simulink model "USMcontrolSystem"  (R2017a)
settings: Solver=FixedStepAuto  StartTime=0.0  StopTime=300  FixedStep=0.01666  RelTol=1e-3
values from neighbouring files (symbols this model uses):
  modelParams = load('usm_params.mat')    [vortex_initializeSimulation.m]
  q_IC = zeros(1,8)    [vortexParameters.m]
  T_cm_cb = [rotationX(pi), [0.09 0 0]'; zeros(1,3), 1]    [vortexParameters.m]
  T_head_front = [rotationX(pi), zeros(3,1); zeros(1,3), 1]    [vortexParameters.m]
  T_I_vx = eye(4)    [vortexParameters.m]
  T_tail_back = [rotationZ(pi) * rotationX(pi), [0.105,0,0]'; zeros(1,3), 1]    [vortexParameters.m]
  T_vx_cm_IC = [rotationZ(pi), [0.240, 0, -180]'; zeros(1,3),1]    [vortexParameters.m]
  T_vx_head_IC = [rotationZ(pi), [-1.371,0,-180]'; zeros(1,3), 1]    [vortexParameters.m]
  T_vx_tail_IC = [eye(3), [1.817,0,-180]'; zeros(1,3), 1]    [vortexParameters.m]
undefined symbols (not defined in the file or in its folder): Ke_D, Ke_P, waypoints
undefined symbols (not defined in the file): thrustAlloc
libraries: powerlib_meascontrol x1, Vortex x1
settings Model: Creator=jorgesv  LastModifiedBy=bjorhho

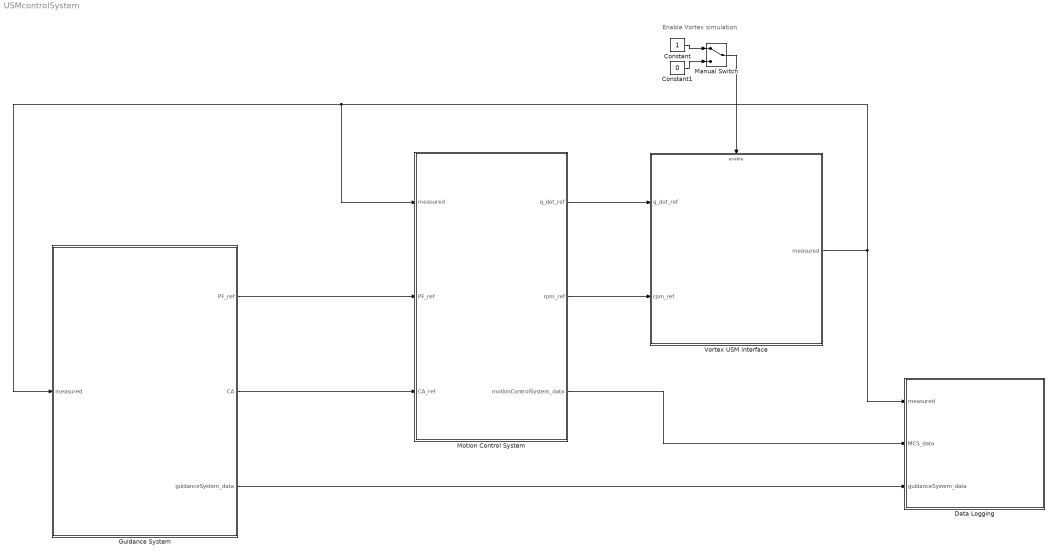
== system USMcontrolSystem ==
  note: Enable Vortex simulation
  Constant : Constant
  Constant1 : Constant  Value=0
  Data Logging : Subsystem
  Guidance System : Subsystem
  Manual Switch : ManualSwitch
  Motion Control System : Subsystem
  Vortex USM interface : Subsystem  TreatAsAtomicUnit=on  mask{T_vx_head_IC=T_vx_head_IC, T_vx_tail_IC=T_vx_tail_IC, q_IC=q_IC, T_0_vx=T_I_vx, T_head_front=T_head_front, T_tail_back=T_tail_back}
      mask prompts: T_vx_head_IC "Transformation from Vortex frame to head module frame"; T_vx_tail_IC "Tronsformation from Vortex frame to tail module frame"; q_IC "Joint positions"; T_0_vx "Transformation from inertial frame to Vortex frame"; T_head_front "Transformation from head module frame to front frame"; T_tail_back "Transformation from tail module frame to back frame"
      settings: MinAlgLoopOccurrences=on
  wires:
  Manual Switch/1 -> Vortex USM interface/Enable
  Constant/1 -> Manual Switch/1
  Constant1/1 -> Manual Switch/2
  Vortex USM interface/1(measured) -> Data Logging/1(measured), Guidance System/1(measured), Motion Control System/1(measured)
  Guidance System/3(guidanceSystem_data) -> Data Logging/3(guidanceSystem_data)
  Guidance System/1(PF_ref) -> Motion Control System/2(PF_ref)
  Motion Control System/2(rpm_ref) -> Vortex USM interface/2(rpm_ref)
  Motion Control System/1(q_dot_ref) -> Vortex USM interface/1(q_dot_ref)
  Motion Control System/3(motionControlSystem_data) -> Data Logging/2(MCS_data)
  Guidance System/2(CA) -> Motion Control System/3(CA_ref)

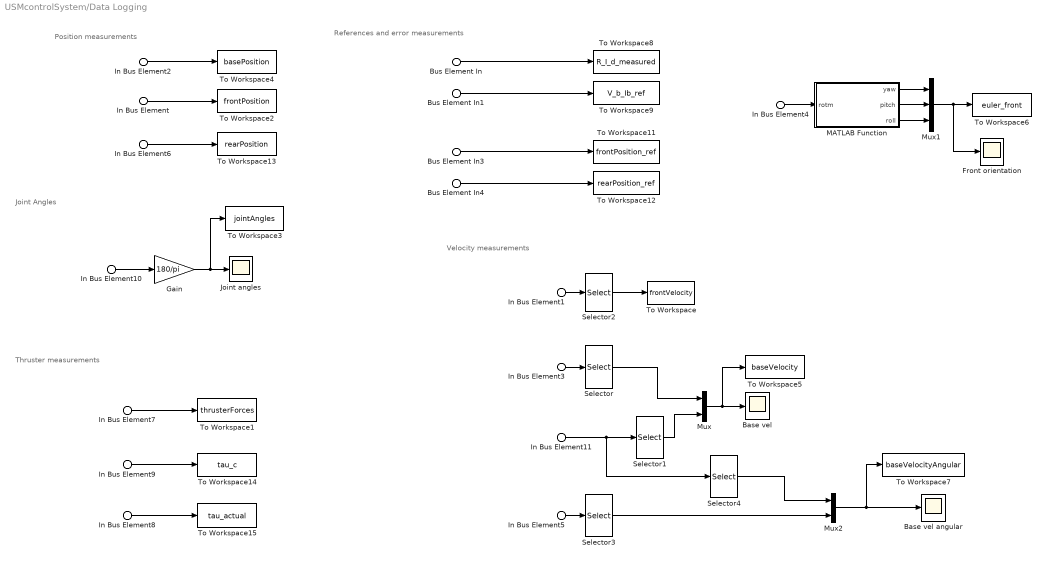
== system USMcontrolSystem/Data Logging ==
  note: References and error measurements
  note: Thruster measurements
  note: Velocity measurements
  note: Position measurements
  note: Joint Angles
  In Bus Element1 : Inport  PortName=measured  Element=V_If_f
  In Bus Element3 : Inport  PortName=measured  Element=V_Ib_b
  In Bus Element5 : Inport  PortName=measured  Element=V_Ib_b
  In Bus Element : Inport  PortName=measured  Element=p_I_f
  In Bus Element2 : Inport  PortName=measured  Element=p_I_b
  In Bus Element4 : Inport  PortName=measured  Element=R_I_f
  In Bus Element6 : Inport  PortName=measured  Element=p_I_r
  In Bus Element10 : Inport  PortName=measured  Element=q_m
  In Bus Element7 : Inport  Port=2  PortName=MCS_data  Element=f_thr
  In Bus Element8 : Inport  Port=2  PortName=MCS_data  Element=actualThrust
  In Bus Element9 : Inport  Port=2  PortName=MCS_data  Element=tau_c
  In Bus Element11 : Inport  Port=2  PortName=MCS_data  Element=V_b_Ib_tilde
  Bus Element In : Inport  Port=3  PortName=guidanceSystem_data  Element=R_I_d
  Bus Element In1 : Inport  Port=3  PortName=guidanceSystem_data  Element=V_b_Ib_tilde
  Bus Element In3 : Inport  Port=3  PortName=guidanceSystem_data  Element=pf_ref
  Bus Element In4 : Inport  Port=3  PortName=guidanceSystem_data  Element=pr_ref
  Base vel : Scope
  Base vel angular : Scope
  Front orientation : Scope
  Gain : Gain  Gain=180/pi
  Joint angles : Scope
  MATLAB Function : MATLAB Function  TreatAsAtomicUnit=on
  Mux : Mux  Inputs=2
  Mux1 : Mux  Inputs=3
  Mux2 : Mux  Inputs=2
  Selector : Selector  InputPortWidth=6  IndexOptions=Index vector (dialog)  Indices=1:3  OutputSizes=1
  Selector1 : Selector  InputPortWidth=6  IndexOptions=Index vector (dialog)  Indices=1:3  OutputSizes=1
  Selector2 : Selector  InputPortWidth=6  IndexOptions=Index vector (dialog)  Indices=1:3  OutputSizes=1
  Selector3 : Selector  InputPortWidth=6  IndexOptions=Index vector (dialog)  Indices=4:6  OutputSizes=1
  Selector4 : Selector  InputPortWidth=6  IndexOptions=Index vector (dialog)  Indices=4:6  OutputSizes=1
  To Workspace : ToWorkspace  VariableName=frontVelocity  SaveFormat=Timeseries  SampleTime=-1
  To Workspace1 : ToWorkspace  VariableName=thrusterForces  SaveFormat=Timeseries  SampleTime=-1
  To Workspace11 : ToWorkspace  VariableName=frontPosition_ref  SaveFormat=Timeseries  SampleTime=-1
  To Workspace12 : ToWorkspace  VariableName=rearPosition_ref  SaveFormat=Timeseries  SampleTime=-1
  To Workspace13 : ToWorkspace  VariableName=rearPosition  SaveFormat=Timeseries  SampleTime=-1
  To Workspace14 : ToWorkspace  VariableName=tau_c  SaveFormat=Timeseries  SampleTime=-1
  To Workspace15 : ToWorkspace  VariableName=tau_actual  SaveFormat=Timeseries  SampleTime=-1
  To Workspace2 : ToWorkspace  VariableName=frontPosition  SaveFormat=Timeseries  SampleTime=-1
  To Workspace3 : ToWorkspace  VariableName=jointAngles  SaveFormat=Timeseries  SampleTime=-1
  To Workspace4 : ToWorkspace  VariableName=basePosition  SaveFormat=Timeseries  SampleTime=-1
  To Workspace5 : ToWorkspace  VariableName=baseVelocity  SaveFormat=Timeseries  SampleTime=-1
  To Workspace6 : ToWorkspace  VariableName=euler_front  SaveFormat=Timeseries  SampleTime=-1
  To Workspace7 : ToWorkspace  VariableName=baseVelocityAngular  SaveFormat=Timeseries  SampleTime=-1
  To Workspace8 : ToWorkspace  VariableName=R_I_d_measured  SaveFormat=Timeseries  SampleTime=-1
  To Workspace9 : ToWorkspace  VariableName=V_b_Ib_ref  SaveFormat=Timeseries  SampleTime=-1
  wires:
  In Bus Element1/1 -> Selector2/1
  In Bus Element3/1 -> Selector/1
  In Bus Element8/1 -> To Workspace15/1
  Selector/1 -> Mux/1
  Selector2/1 -> To Workspace/1
  Gain/1 -> To Workspace3/1, Joint angles/1
  Mux/1 -> To Workspace5/1, Base vel/1
  In Bus Element4/1 -> MATLAB Function/1(rotm)
  MATLAB Function/1(yaw) -> Mux1/1
  MATLAB Function/2(pitch) -> Mux1/2
  MATLAB Function/3(roll) -> Mux1/3
  Mux1/1 -> Front orientation/1, To Workspace6/1
  In Bus Element/1 -> To Workspace2/1
  In Bus Element2/1 -> To Workspace4/1
  Selector1/1 -> Mux/2
  Mux2/1 -> To Workspace7/1, Base vel angular/1
  In Bus Element5/1 -> Selector3/1
  In Bus Element11/1 -> Selector4/1, Selector1/1
  Bus Element In/1 -> To Workspace8/1
  Bus Element In1/1 -> To Workspace9/1
  Bus Element In3/1 -> To Workspace11/1
  Bus Element In4/1 -> To Workspace12/1
  In Bus Element6/1 -> To Workspace13/1
  Selector4/1 -> Mux2/1
  Selector3/1 -> Mux2/2
  In Bus Element7/1 -> To Workspace1/1
  In Bus Element9/1 -> To Workspace14/1
  In Bus Element10/1 -> Gain/1

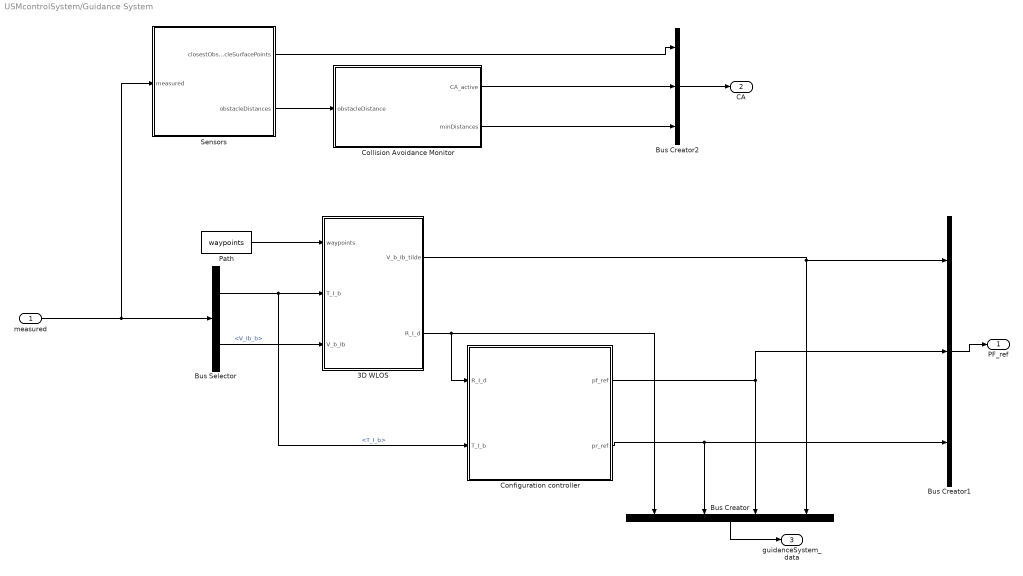
== system USMcontrolSystem/Guidance System ==
  measured : Inport
  3D WLOS : MATLAB Function  TreatAsAtomicUnit=on
  Bus Creator : BusCreator  Inputs=4
  Bus Creator1 : BusCreator  Inputs=3
  Bus Creator2 : BusCreator  Inputs=3
  Bus Selector : BusSelector  OutputSignals=T_I_b,V_Ib_b
  Collision Avoidance Monitor : MATLAB Function  TreatAsAtomicUnit=on
  Configuration controller : MATLAB Function  TreatAsAtomicUnit=on
  Path : Constant  Value=waypoints  VectorParams1D=off
  Sensors : Subsystem
  PF_ref : Outport
  CA : Outport  Port=2
  guidanceSystem_data : Outport  Port=3
  wires:
  Path/1 -> 3D WLOS/1(waypoints)
  3D WLOS/2(R_I_d) -> Configuration controller/1(R_I_d), Bus Creator/1
  Configuration controller/1(pf_ref) -> Bus Creator1/2, Bus Creator/3
  Configuration controller/2(pr_ref) -> Bus Creator/2, Bus Creator1/3
  Bus Creator/1 -> guidanceSystem_data/1
  Bus Creator1/1 -> PF_ref/1
  measured/1 -> Sensors/1(measured), Bus Selector/1
  Bus Selector/1 -> Configuration controller/2(T_I_b), 3D WLOS/2(T_I_b)  "<T_I_b>"
  Bus Selector/2 -> 3D WLOS/3(V_b_Ib)  "<V_Ib_b>"
  Sensors/2(obstacleDistances) -> Collision Avoidance Monitor/1(obstacleDistance)
  Collision Avoidance Monitor/1(CA_active) -> Bus Creator2/2
  Sensors/1(closestObstacleSurfacePoints) -> Bus Creator2/1
  Bus Creator2/1 -> CA/1
  Collision Avoidance Monitor/2(minDistances) -> Bus Creator2/3
  3D WLOS/1(V_b_Ib_tilde) -> Bus Creator/4, Bus Creator1/1

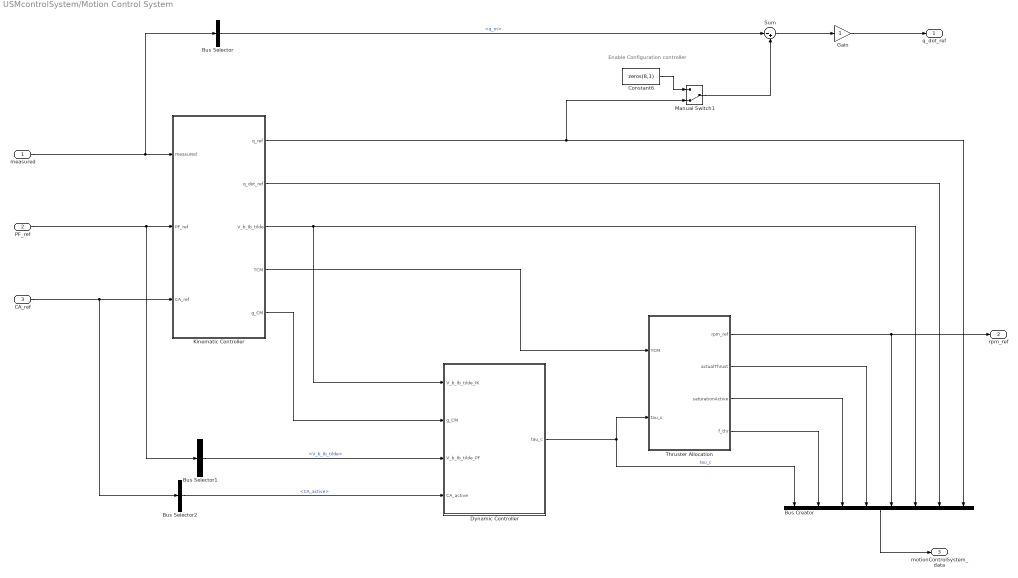
== system USMcontrolSystem/Motion Control System ==
  note: Enable Configuration controller
  measured : Inport
  PF_ref : Inport  Port=2
  CA_ref : Inport  Port=3
  Bus Creator : BusCreator  Inputs=8
  Bus Selector : BusSelector  OutputSignals=q_m
  Bus Selector1 : BusSelector  OutputSignals=V_b_Ib_tilde
  Bus Selector2 : BusSelector  OutputSignals=CA_active
  Constant6 : Constant  Value=zeros(8,1)
  Dynamic Controller : Subsystem
  Gain : Gain
  Kinematic Controller : Subsystem
  Manual Switch1 : ManualSwitch  CurrentSetting=0
  Sum : Sum  Inputs=|-+
  Thruster Allocation : Subsystem  mask{W=thrustAlloc.W_thr, Q_inv=thrustAlloc.Q_thr_inv, mode=thrustAlloc.mode}
      mask prompts: W "Thruster weights"; Q_inv "Pseudoinverse damping matrix (Q_inv)"; mode "Thrust allocation mode"
  q_dot_ref : Outport
  rpm_ref : Outport  Port=2
  motionControlSystem_data : Outport  Port=3
  wires:
  PF_ref/1 -> Bus Selector1/1, Kinematic Controller/2(PF_ref)
  measured/1 -> Bus Selector/1, Kinematic Controller/1(measured)
  Bus Selector/1 -> Sum/1  "<q_m>"
  Dynamic Controller/1(tau_c) -> Thruster Allocation/2(tau_c), Bus Creator/1  "tau_c"
  Thruster Allocation/1(rpm_ref) -> rpm_ref/1, Bus Creator/5
  Bus Creator/1 -> motionControlSystem_data/1
  Thruster Allocation/4(f_thr) -> Bus Creator/2
  Thruster Allocation/3(saturationActive) -> Bus Creator/3
  Thruster Allocation/2(actualThrust) -> Bus Creator/4
  Sum/1 -> Gain/1
  Gain/1 -> q_dot_ref/1
  Manual Switch1/1 -> Sum/2
  Constant6/1 -> Manual Switch1/1
  Kinematic Controller/3(V_b_Ib_tilde) -> Dynamic Controller/1(V_b_Ib_tilde_IK), Bus Creator/6
  CA_ref/1 -> Bus Selector2/1, Kinematic Controller/3(CA_ref)
  Bus Selector2/1 -> Dynamic Controller/4(CA_active)  "<CA_active>"
  Kinematic Controller/2(q_dot_ref) -> Bus Creator/7
  Kinematic Controller/1(q_ref) -> Manual Switch1/2, Bus Creator/8
  Bus Selector1/1 -> Dynamic Controller/3(V_b_Ib_tilde_PF)  "<V_b_Ib_tilde>"
  Kinematic Controller/5(g_CM) -> Dynamic Controller/2(g_CM)
  Kinematic Controller/4(TCM) -> Thruster Allocation/1(TCM)

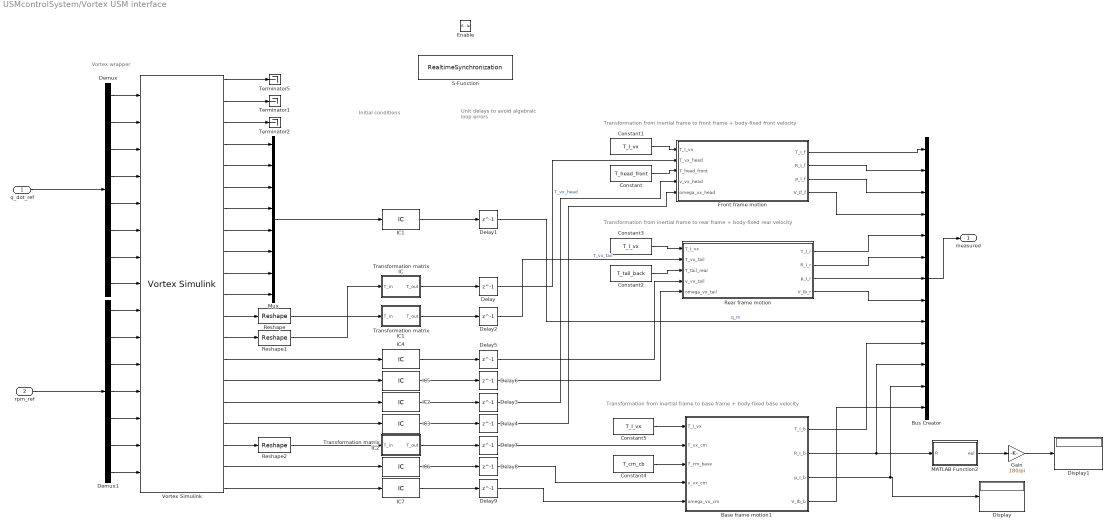
== system USMcontrolSystem/Vortex USM interface ==
  note: Initial conditions
  note: Unit delays to avoid
      | algebraic loop errors
  note: Transformation from inertial frame to front frame + body-fixed front velocity
  note: Vortex wrapper
  note: Transformation from inertial frame to rear frame + body-fixed rear velocity
  note: Transformation from inertial frame to base frame + body-fixed base velocity
  q_dot_ref : Inport  Unit=rad
  rpm_ref : Inport  Port=2  Unit=rpm
  Enable : EnablePort
  Base frame motion1 : MATLAB Function  TreatAsAtomicUnit=on
  Bus Creator : BusCreator  Inputs=13
  Constant : Constant  Value=T_head_front
  Constant1 : Constant  Value=T_I_vx
  Constant2 : Constant  Value=T_tail_back
  Constant3 : Constant  Value=T_I_vx
  Constant4 : Constant  Value=T_cm_cb
  Constant5 : Constant  Value=T_I_vx
  Delay : Delay  DelayLength=1  InitialCondition=T_vx_head_IC
  Delay1 : Delay  DelayLength=1  InitialCondition=q_IC
  Delay2 : Delay  DelayLength=1  InitialCondition=T_vx_tail_IC
  Delay{3..6,8..9} (6 alike) : Delay  DelayLength=1  InitialCondition=[0,0,0]'
  Delay7 : Delay  DelayLength=1  InitialCondition=T_vx_cm_IC
  Demux : Demux  Outputs=8
  Demux1 : Demux  Outputs=7
  Display : Display
  Display1 : Display
  Front frame motion : MATLAB Function  TreatAsAtomicUnit=on
  Gain : Gain  Gain=180/pi
  IC1 : InitialCondition  Value=q_IC
  IC{2..7} (6 alike) : InitialCondition  Value=[0,0,0]'
  MATLAB Function2 : MATLAB Function  TreatAsAtomicUnit=on
  Mux : Mux  Inputs=8
  Rear frame motion : MATLAB Function  TreatAsAtomicUnit=on
  Reshape : Reshape  OutputDimensionality=Customize  OutputDimensions=[4,4]
  Reshape1 : Reshape  OutputDimensionality=Customize  OutputDimensions=[4,4]
  Reshape2 : Reshape  OutputDimensionality=Customize  OutputDimensions=[4,4]
  S-Function : S-Function  FunctionName=RealtimeSynchronization  SFunctionDeploymentMode=off  EnableBusSupport=off
  Terminator1 : Terminator
  Terminator2 : Terminator
  Terminator5 : Terminator
  Transformation matrix IC : Subsystem  mask{T_init=T_vx_head_IC}
      mask prompts: T_init "Initial condition"
      mask DialogControl DescTextVar Prompt: Outputs T_init when T_in is an invalid transformation matrix. Outputs T_in when it is valid.
  Transformation matrix IC1 : Subsystem  mask{T_init=T_vx_tail_IC}
      mask prompts: T_init "Initial condition"
      mask DialogControl DescTextVar Prompt: Outputs T_init when T_in is an invalid transformation matrix. Outputs T_in when it is valid.
  Transformation matrix IC2 : Subsystem  mask{T_init=T_vx_cm_IC}
      mask prompts: T_init "Initial condition"
      mask DialogControl DescTextVar Prompt: Outputs T_init when T_in is an invalid transformation matrix. Outputs T_in when it is valid.
  Vortex Simulink : Vortex/Vortex Simulink  ip='127.0.0.1'  port='736'  path='C:\Users\bjorhho\Google Drive\Skole\NTNU\Masteroppgave\Vortex\Source code\Control System\Vortex-Simulink-interface-velocity.json'  display=image(imread('logo.jpg'), [0, 0, 48, 48]);fprintf('\n\n\nMy Model');port_label('input',1,'q1_cmd');port_label('input',2,'q2_cmd');port_label('input',3,'q3_cmd');port_label('input',4,'q4_cmd');port_label('input',5,'q5_cmd');port_label('input',6,'q6_cmd');port_label('input',7,'q7_cmd');port_label('input',8,'q8_cmd');port_label('input',9,'u1_rpm');port_label('input',10,'u2_rpm');port_label('input',11,'u3_rpm');port_label('input',12,'u4_rpm');port_label('input',13,'u5_rpm');port_label('input',14,'u6_rpm');port_label('input',15,'u7_rpm');port_label('output',1,'Status');port_label('output',2,'Time');port_label('output',3,'FrameIndex');port_label('output',4,'q1');port_label('output',5,'q2');port_label('output',6,'q3');port_label('output',7,'q4');port_label('output',8,'q5');port_label('output',9,'q6');port_label('output',10,'q7');port_label('output',11,'q8');port_label('output',12,'T_vx_tail');port_label('output',13,'T_vx_head');port_label('output',14,'v_vx_tail');port_label('output',15,'w_vx_tail');port_label('output',16,'v_vx_head');port_label('output',17,'w_vx_head');port_label('output',18,'T_vx_cm');port_label('output',19,'v_vx_cm');port_label('output',20,'w_vx_cm');  SynchronizationMechanism=None  WaitVortex=off
      settings: SourceProductName=Vortex
  measured : Outport
  wires:
  Vortex Simulink/17 -> IC3/1
  Vortex Simulink/16 -> IC2/1
  Vortex Simulink/15 -> IC5/1
  Vortex Simulink/14 -> IC4/1
  Reshape/1 -> Transformation matrix IC1/1(T_in)
  Reshape1/1 -> Transformation matrix IC/1(T_in)
  Vortex Simulink/13 -> Reshape1/1
  Vortex Simulink/12 -> Reshape/1
  Vortex Simulink/11 -> Mux/8
  Vortex Simulink/10 -> Mux/7
  Vortex Simulink/9 -> Mux/6
  Vortex Simulink/8 -> Mux/5
  Vortex Simulink/7 -> Mux/4
  Vortex Simulink/6 -> Mux/3
  Vortex Simulink/5 -> Mux/2
  Vortex Simulink/4 -> Mux/1
  Mux/1 -> IC1/1
  Demux1/6 -> Vortex Simulink/14
  Demux1/1 -> Vortex Simulink/9
  Demux1/4 -> Vortex Simulink/12
  Demux1/5 -> Vortex Simulink/13
  Demux1/7 -> Vortex Simulink/15
  Demux1/3 -> Vortex Simulink/11
  Demux1/2 -> Vortex Simulink/10
  Vortex Simulink/1 -> Terminator5/1
  Demux/8 -> Vortex Simulink/8
  Demux/7 -> Vortex Simulink/7
  Demux/6 -> Vortex Simulink/6
  Demux/5 -> Vortex Simulink/5
  Demux/4 -> Vortex Simulink/4
  Demux/3 -> Vortex Simulink/3
  Demux/2 -> Vortex Simulink/2
  Demux/1 -> Vortex Simulink/1
  Vortex Simulink/2 -> Terminator1/1
  Vortex Simulink/3 -> Terminator2/1
  IC1/1 -> Delay1/1
  Delay1/1 -> Bus Creator/9  "q_m"
  Bus Creator/1 -> measured/1
  Constant3/1 -> Rear frame motion/1(T_I_vx)
  Constant2/1 -> Rear frame motion/3(T_tail_rear)
  Constant1/1 -> Front frame motion/1(T_I_vx)
  Front frame motion/1(T_I_f) -> Bus Creator/1
  Front frame motion/2(R_I_f) -> Bus Creator/2
  Front frame motion/4(V_If_f) -> Bus Creator/4
  Delay3/1 -> Front frame motion/4(v_vx_head)
  Constant/1 -> Front frame motion/3(T_head_front)
  Delay/1 -> Front frame motion/2(T_vx_head)  "T_vx_head"
  Delay4/1 -> Front frame motion/5(omega_vx_head)
  Front frame motion/3(p_I_f) -> Bus Creator/3
  MATLAB Function2/1(eul) -> Gain/1
  IC3/1 -> Delay4/1
  IC2/1 -> Delay3/1
  IC5/1 -> Delay6/1
  IC4/1 -> Delay5/1
  Transformation matrix IC1/1(T_out) -> Delay2/1
  Transformation matrix IC/1(T_out) -> Delay/1
  Vortex Simulink/18 -> Reshape2/1
  Vortex Simulink/20 -> IC7/1
  Vortex Simulink/19 -> IC6/1
  Reshape2/1 -> Transformation matrix IC2/1(T_in)
  Transformation matrix IC2/1(T_out) -> Delay7/1
  IC6/1 -> Delay8/1
  IC7/1 -> Delay9/1
  Constant4/1 -> Base frame motion1/3(T_cm_base)
  Constant5/1 -> Base frame motion1/1(T_I_vx)
  Delay7/1 -> Base frame motion1/2(T_vx_cm)
  Delay8/1 -> Base frame motion1/4(v_vx_cm)
  Delay9/1 -> Base frame motion1/5(omega_vx_cm)
  Rear frame motion/4(V_Ib_r) -> Bus Creator/8
  Rear frame motion/3(p_I_r) -> Bus Creator/7
  Rear frame motion/2(R_I_r) -> Bus Creator/6
  Rear frame motion/1(T_I_r) -> Bus Creator/5
  Delay2/1 -> Rear frame motion/2(T_vx_tail)  "T_vx_tail"
  Delay5/1 -> Rear frame motion/4(v_vx_tail)
  Delay6/1 -> Rear frame motion/5(omega_vx_tail)
  Base frame motion1/2(R_I_b) -> Bus Creator/11, MATLAB Function2/1(R)
  Base frame motion1/3(p_I_b) -> Bus Creator/12, Display/1
  Gain/1 -> Display1/1
  rpm_ref/1 -> Demux1/1
  Base frame motion1/1(T_I_b) -> Bus Creator/10
  Base frame motion1/4(V_Ib_b) -> Bus Creator/13
  q_dot_ref/1 -> Demux/1

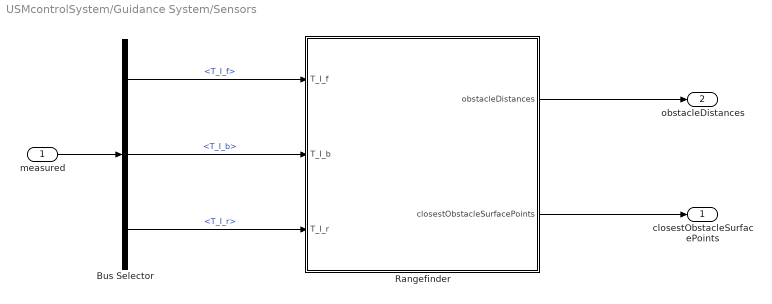
== system USMcontrolSystem/Guidance System/Sensors ==
  measured : Inport
  Bus Selector : BusSelector  OutputSignals=T_I_f,T_I_b,T_I_r
  Rangefinder : MATLAB Function  TreatAsAtomicUnit=on
  closestObstacleSurfacePoints : Outport
  obstacleDistances : Outport  Port=2
  wires:
  measured/1 -> Bus Selector/1
  Bus Selector/1 -> Rangefinder/1(T_I_f)  "<T_I_f>"
  Bus Selector/2 -> Rangefinder/2(T_I_b)  "<T_I_b>"
  Bus Selector/3 -> Rangefinder/3(T_I_r)  "<T_I_r>"
  Rangefinder/1(obstacleDistances) -> obstacleDistances/1
  Rangefinder/2(closestObstacleSurfacePoints) -> closestObstacleSurfacePoints/1

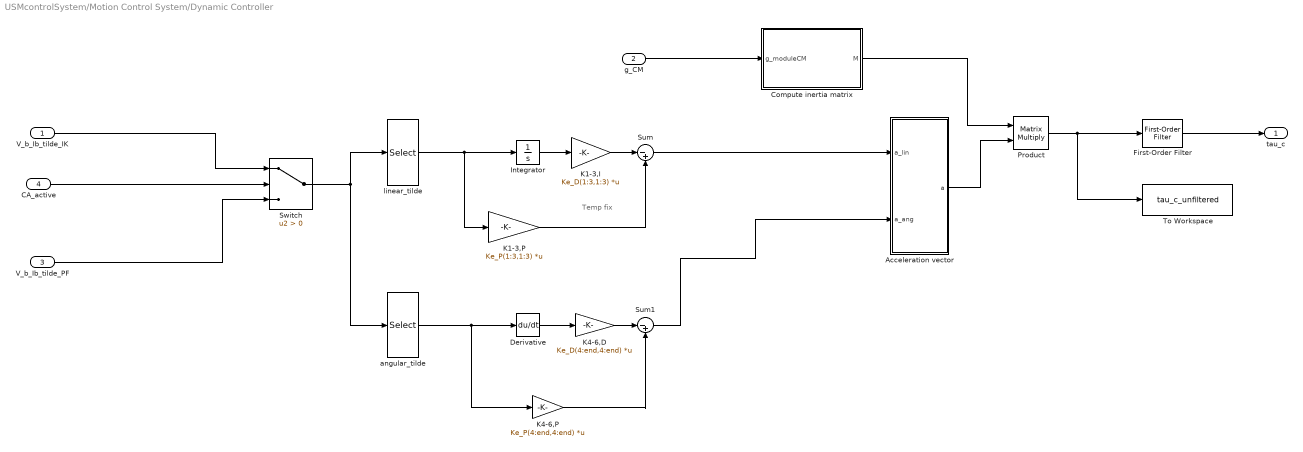
== system USMcontrolSystem/Motion Control System/Dynamic Controller ==
  note: Temp fix
  V_b_Ib_tilde_IK : Inport
  g_CM : Inport  Port=2
  V_b_Ib_tilde_PF : Inport  Port=3
  CA_active : Inport  Port=4
  Acceleration vector : MATLAB Function  TreatAsAtomicUnit=on
  Compute inertia matrix : MATLAB Function  TreatAsAtomicUnit=on
  Derivative : Derivative
  First-Order Filter : powerlib_meascontrol/Filters/First-Order Filter  FilterType=Lowpass  Tc=0.1  Ts=0  Initialize=on  Vac_Init=[0, 0, 60]  Vdc_Init=0  PlotResponse=off  FreqRange="[0,  200,  1]"
      settings: SourceProductName=Simscape Power Systems
  Integrator : Integrator
  K1-3,I : Gain  Gain=Ke_D(1:3,1:3)  Multiplication=Matrix(K*u)
  K1-3,P : Gain  Gain=Ke_P(1:3,1:3)  Multiplication=Matrix(K*u)
  K4-6,D : Gain  Gain=Ke_D(4:end,4:end)  Multiplication=Matrix(K*u)
  K4-6,P : Gain  Gain=Ke_P(4:end,4:end)  Multiplication=Matrix(K*u)
  Product : Product  Multiplication=Matrix(*)
  Sum : Sum  Inputs=|-+
  Sum1 : Sum  Inputs=|-+
  Switch : Switch  Criteria=u2 > Threshold
  To Workspace : ToWorkspace  VariableName=tau_c_unfiltered  SaveFormat=Timeseries  SampleTime=-1
  angular_tilde : Selector  InputPortWidth=6  IndexOptions=Index vector (dialog)  Indices=[4 5 6]  OutputSizes=1
  linear_tilde : Selector  InputPortWidth=6  IndexOptions=Index vector (dialog)  Indices=[1 2 3]  OutputSizes=1
  tau_c : Outport
  wires:
  g_CM/1 -> Compute inertia matrix/1(g_moduleCM)
  Compute inertia matrix/1(M) -> Product/1
  Integrator/1 -> K1-3,I/1
  K1-3,I/1 -> Sum/1
  Derivative/1 -> K4-6,D/1
  K4-6,D/1 -> Sum1/1
  K4-6,P/1 -> Sum1/2
  Sum/1 -> Acceleration vector/1(a_lin)
  Sum1/1 -> Acceleration vector/2(a_ang)
  Acceleration vector/1(a) -> Product/2
  Product/1 -> First-Order Filter/1, To Workspace/1
  First-Order Filter/1 -> tau_c/1
  V_b_Ib_tilde_PF/1 -> Switch/3
  Switch/1 -> angular_tilde/1, linear_tilde/1
  linear_tilde/1 -> K1-3,P/1, Integrator/1
  angular_tilde/1 -> K4-6,P/1, Derivative/1
  K1-3,P/1 -> Sum/2
  CA_active/1 -> Switch/2
  V_b_Ib_tilde_IK/1 -> Switch/1

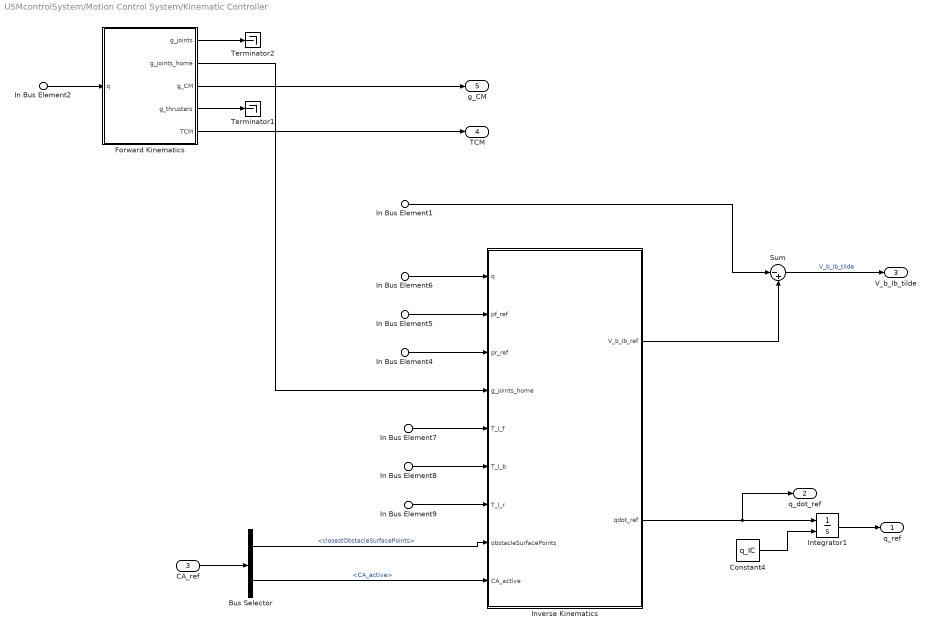
== system USMcontrolSystem/Motion Control System/Kinematic Controller ==
  In Bus Element9 : Inport  PortName=measured  Element=T_I_r
  In Bus Element7 : Inport  PortName=measured  Element=T_I_f
  In Bus Element8 : Inport  PortName=measured  Element=T_I_b
  In Bus Element6 : Inport  PortName=measured  Element=q_m
  In Bus Element2 : Inport  PortName=measured  Element=q_m
  In Bus Element1 : Inport  PortName=measured  Element=V_Ib_b
  In Bus Element4 : Inport  Port=2  PortName=PF_ref  Element=pr_ref
  In Bus Element5 : Inport  Port=2  PortName=PF_ref  Element=pf_ref
  CA_ref : Inport  Port=3
  Bus Selector : BusSelector  OutputSignals=closestObstacleSurfacePoints,CA_active
  Constant4 : Constant  Value=q_IC
  Forward Kinematics : Subsystem
  Integrator1 : Integrator  InitialConditionSource=external  InitialCondition=q_IC
  Inverse Kinematics : MATLAB Function  TreatAsAtomicUnit=on
  Sum : Sum  Inputs=|-+
  Terminator1 : Terminator
  Terminator2 : Terminator
  q_ref : Outport
  q_dot_ref : Outport  Port=2
  V_b_Ib_tilde : Outport  Port=3
  TCM : Outport  Port=4
  g_CM : Outport  Port=5
  wires:
  Forward Kinematics/2(g_joints_home) -> Inverse Kinematics/4(g_joints_home)
  In Bus Element7/1 -> Inverse Kinematics/5(T_I_f)
  In Bus Element8/1 -> Inverse Kinematics/6(T_I_b)
  In Bus Element9/1 -> Inverse Kinematics/7(T_I_r)
  Bus Selector/1 -> Inverse Kinematics/8(obstacleSurfacePoints)  "<closestObstacleSurfacePoints>"
  Constant4/1 -> Integrator1/2
  Inverse Kinematics/2(qdot_ref) -> q_dot_ref/1, Integrator1/1
  Integrator1/1 -> q_ref/1
  CA_ref/1 -> Bus Selector/1
  Bus Selector/2 -> Inverse Kinematics/9(CA_active)  "<CA_active>"
  In Bus Element5/1 -> Inverse Kinematics/2(pf_ref)
  In Bus Element4/1 -> Inverse Kinematics/3(pr_ref)
  In Bus Element6/1 -> Inverse Kinematics/1(q)
  In Bus Element1/1 -> Sum/1
  Inverse Kinematics/1(V_b_Ib_ref) -> Sum/2
  Sum/1 -> V_b_Ib_tilde/1  "V_b_Ib_tilde"
  Forward Kinematics/5(TCM) -> TCM/1
  Forward Kinematics/3(g_CM) -> g_CM/1
  Forward Kinematics/4(g_thrusters) -> Terminator1/1
  Forward Kinematics/1(g_joints) -> Terminator2/1
  In Bus Element2/1 -> Forward Kinematics/1(q)

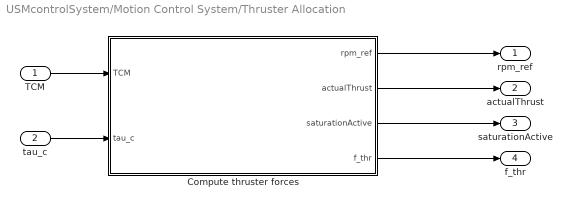
== system USMcontrolSystem/Motion Control System/Thruster Allocation ==
  TCM : Inport
  tau_c : Inport  Port=2
  Compute thruster forces : MATLAB Function  TreatAsAtomicUnit=on
  rpm_ref : Outport
  actualThrust : Outport  Port=2
  saturationActive : Outport  Port=3
  f_thr : Outport  Port=4
  wires:
  Compute thruster forces/1(rpm_ref) -> rpm_ref/1
  TCM/1 -> Compute thruster forces/1(TCM)
  tau_c/1 -> Compute thruster forces/2(tau_c)
  Compute thruster forces/3(saturationActive) -> saturationActive/1
  Compute thruster forces/2(actualThrust) -> actualThrust/1
  Compute thruster forces/4(f_thr) -> f_thr/1

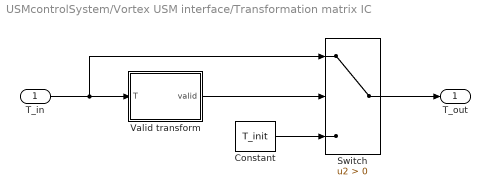
== system USMcontrolSystem/Vortex USM interface/Transformation matrix IC ==
  T_in : Inport
  Constant : Constant  Value=T_init
  Switch : Switch  Criteria=u2 > Threshold
  Valid transform : MATLAB Function  TreatAsAtomicUnit=on
  T_out : Outport
  wires:
  Valid transform/1(valid) -> Switch/2
  T_in/1 -> Switch/1, Valid transform/1(T)
  Constant/1 -> Switch/3
  Switch/1 -> T_out/1

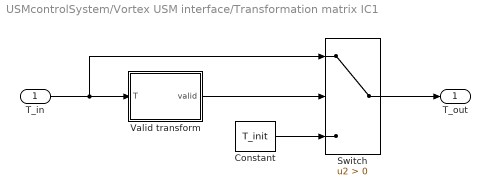
== system USMcontrolSystem/Vortex USM interface/Transformation matrix IC1 ==
  T_in : Inport
  Constant : Constant  Value=T_init
  Switch : Switch  Criteria=u2 > Threshold
  Valid transform : MATLAB Function  TreatAsAtomicUnit=on
  T_out : Outport
  wires:
  Valid transform/1(valid) -> Switch/2
  T_in/1 -> Switch/1, Valid transform/1(T)
  Constant/1 -> Switch/3
  Switch/1 -> T_out/1

== system USMcontrolSystem/Vortex USM interface/Transformation matrix IC2 ==
  T_in : Inport
  Constant : Constant  Value=T_init
  Switch : Switch  Criteria=u2 > Threshold
  Valid transform : MATLAB Function  TreatAsAtomicUnit=on
  T_out : Outport
  wires:
  Switch/1 -> T_out/1
  Constant/1 -> Switch/3
  T_in/1 -> Valid transform/1(T), Switch/1
  Valid transform/1(valid) -> Switch/2

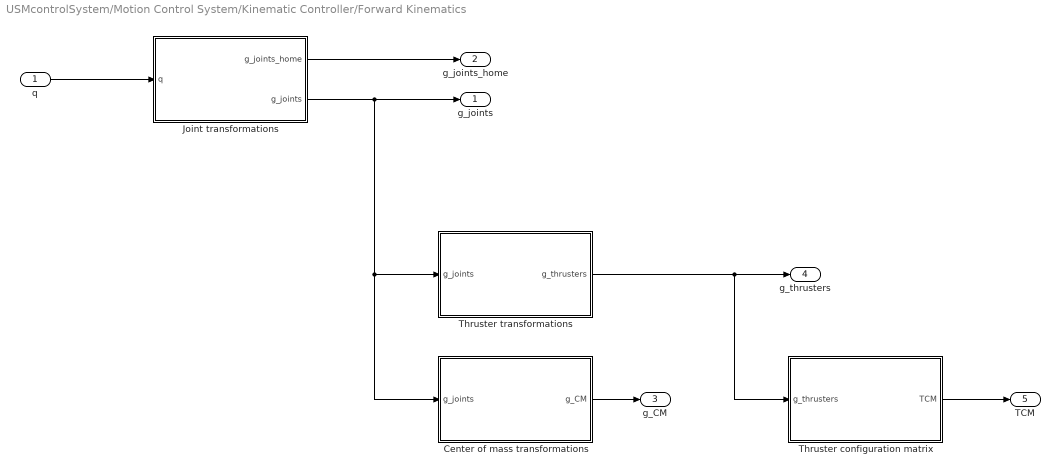
== system USMcontrolSystem/Motion Control System/Kinematic Controller/Forward Kinematics ==
  q : Inport
  Center of mass transformations : MATLAB Function  TreatAsAtomicUnit=on
  Joint transformations : MATLAB Function  TreatAsAtomicUnit=on
  Thruster configuration matrix : MATLAB Function  TreatAsAtomicUnit=on
  Thruster transformations : MATLAB Function  TreatAsAtomicUnit=on
  g_joints : Outport
  g_joints_home : Outport  Port=2
  g_CM : Outport  Port=3
  g_thrusters : Outport  Port=4
  TCM : Outport  Port=5
  wires:
  q/1 -> Joint transformations/1(q)
  Joint transformations/2(g_joints) -> Center of mass transformations/1(g_joints), Thruster transformations/1(g_joints), g_joints/1
  Thruster transformations/1(g_thrusters) -> Thruster configuration matrix/1(g_thrusters), g_thrusters/1
  Center of mass transformations/1(g_CM) -> g_CM/1
  Joint transformations/1(g_joints_home) -> g_joints_home/1
  Thruster configuration matrix/1(TCM) -> TCM/1

== matlab function USMcontrolSystem/Motion Control System/Kinematic Controller/Forward Kinematics/Thruster transformations ==
  data: g_joints input; g_thrusters output; modelParams parameter
function g_thrusters = thrusterTransformations(g_joints, modelParams)
%#codegen

% Compute transformations from the joint frames to the thruster frames

num_thrusters = modelParams.num_thrusters;
thruster_ax = modelParams.thruster_ax;
thruster_pos = modelParams.thruster_pos;
thruster_moduleNumber = modelParams.thruster_moduleNumber;

g_thrusters = calculateThrusterTransformations(g_joints, num_thrusters, thruster_ax, thruster_pos, thruster_moduleNumber);

%NEW
%thruster_rotation = modelParams.thruster_rotation;
%g_thrusters = calculateThrusterTransformations(g_joints, num_thrusters, thruster_rotation, thruster_pos, thruster_moduleNumber);

end

== matlab function USMcontrolSystem/Motion Control System/Kinematic Controller/Forward Kinematics/Joint transformations ==
  data: g_joints_home output; q input; g_joints output; modelParams parameter
function [g_joints_home, g_joints] = jointTransformations(q, modelParams)
%#codegen

% Compute transformations from the back frame to each joint frame and to the front (end-effector) frame

num_joints = modelParams.num_joints;
joint_tr = modelParams.joint_tr;
joint_ax = modelParams.joint_ax;

[g_joints, g_joints_home] = calculateJointTransformations(q, num_joints, joint_tr, joint_ax);

end

== matlab function USMcontrolSystem/Guidance System/Sensors/Rangefinder ==
  data: obstacleDistances output; T_I_f input; closestObstacleSurfacePoints output; T_I_b input; T_I_r input
function [obstacleDistances, closestObstacleSurfacePoints] = distanceToObstacles(T_I_f, T_I_b, T_I_r)
persistent obstacles;
if isempty(obstacles)
    %Obstacle course: (the one used in the thesis)
    %Vertical cyldinders
    R_cyl = 0.5;
    d_circ = sqrt(2);
    c_circ = -7;
    c1 = Cylinder([c_circ + d_circ; -d_circ; -185], [c_circ + d_circ; -d_circ; -175], R_cyl);
    c2 = Cylinder([c_circ + d_circ; d_circ; -185], [c_circ + d_circ; d_circ; -175], R_cyl);

    c3 = Cylinder([c_circ; 0.1; -185], [c_circ; 0.1; -175], R_cyl);

    c4 = Cylinder([c_circ - d_circ; -d_circ; -185], [c_circ - d_circ; -d_circ; -175], R_cyl);
    c5 = Cylinder([c_circ - d_circ; d_circ; -185], [c_circ - d_circ; d_circ; -175], R_cyl);
    %Horizontal cylinders
    c6 = Cylinder([c_circ + d_circ; -d_circ; -180.1], [c_circ + d_circ; d_circ; -180.1], R_cyl);
    c7 = Cylinder([c_circ; 0.1; -179], [c_circ - d_circ; -d_circ + 0.1; -179], R_cyl);
    c8 = Cylinder([c_circ - d_circ; -d_circ; -181], [c_circ - d_circ; d_circ; -181], R_cyl);

    obstacles = {c1, c2, c3, c4, c5, c6, c7, c8};
end

p_I_f = tform2trvec(T_I_f);
p_I_b = tform2trvec(T_I_b);
p_I_r = tform2trvec(T_I_r);

nCAPoints = 3;
%obstacles is a cell array containing obstacles as basic shape objects
nObstacles = numel(obstacles);

obstacleDistances = zeros(nCAPoints, nObstacles);
obstacleSurfacePoints = zeros(3, nCAPoints, nObstacles);
CAPoints = [p_I_f p_I_b p_I_r];

closest = Inf(1, nCAPoints);
closestObstacleSurfacePoints = zeros(3, nCAPoints);
for i = 1:nObstacles
    o = obstacles{i};
    for j = 1:nCAPoints
        obstacleDistances(j, i) = o.distanceTo(CAPoints(:,j));
        obstacleSurfacePoints(:,j,i) = o.closestSurfacePointTo(CAPoints(:,j));
        
        if obstacleDistances(j, i) < closest(j)
            closest(j) = obstacleDistances(j, i);
            closestObstacleSurfacePoints(:,j) = obstacleSurfacePoints(:,j,i);
        end
    end
end

end

== matlab function USMcontrolSystem/Motion Control System/Kinematic Controller/Forward Kinematics/Center of mass transformations ==
  data: g_joints input; g_CM output; modelParams parameter
function g_CM = CMTransformations(g_joints, modelParams)
%#codegen

% Compute transformations from the joint frames to the frames attached to
% center of mass of the modules


num_modules = modelParams.num_modules;
module_cm = modelParams.module_cm;

g_CM = calculateModuleTransformations(g_joints, num_modules, module_cm);

end

== matlab function USMcontrolSystem/Motion Control System/Thruster Allocation/Compute thruster forces ==
  data: TCM input; rpm_ref output; actualThrust output; tau_c input; modelParams parameter; W parameter; saturationActive output; f_thr output; Q_inv parameter; mode parameter
function [rpm_ref, actualThrust, saturationActive, f_thr] = distributeThrusterForces(TCM, tau_c, modelParams, W, Q_inv, mode)
%#codegen

n_thr = modelParams.num_thrusters;
thrusterRPMMapping = modelParams.thrusterRPMMapping;

%W = controlParams.W_thr;
%Q_inv = controlParams.Q_thr_inv;
%mode = controlParams.thrustAllocationMode;




% Calculates the distribution of the thruster forces
W_inv = diag(1./diag(W));

switch mode
    case 0   % Standard damped inverse TCM
        [TCM_inv] = calculateTCMInverse(TCM, Q_inv);
        
        [f_thr] = calculateThrusterForces(TCM_inv, tau_c);
        
    case 1   % Thrust allocation with prioritized linear motion (DOF 1-3)
        [TCM_inv_linear,TCM_inv_angular] = calculateTCMInversePrioritized(TCM, Q_inv);
        
        TCM_inv = [TCM_inv_linear, TCM_inv_angular];
        
        [f_thr] = calculateThrusterForcesPrioritized(TCM(1:3,:),TCM_inv_linear,TCM_inv_angular, tau_c, n_thr);
    
    case 2   % Thrust allocation with inverse TCM using SVD
        TCM_inv = calculateTCMInverseSVD(TCM,0.1);
        [f_thr] = calculateThrusterForces(TCM_inv, tau_c);
        
    otherwise  % Equal to case 0
        [TCM_inv] = calculateTCMInverse(TCM, Q_inv);
        
        [f_thr] = calculateThrusterForces(TCM_inv, tau_c);        
end

actualThrust = TCM * f_thr;

mx = max(thrusterRPMMapping(:,2));
mn = min(thrusterRPMMapping(:,2));


% Min/max force saturation to avoid NaN in the RPM interpolation
saturationActive = ~isempty(find(f_thr > mx,1)) + ~isempty(find(f_thr < mn,1));
f_thr(f_thr > mx) = mx;
f_thr(f_thr < mn) = mn;


% Calculate the required RPM
rpm_ref = interp1(thrusterRPMMapping(:,2), thrusterRPMMapping(:,1), f_thr);

end

== matlab function USMcontrolSystem/Guidance System/Collision Avoidance Monitor ==
  data: obstacleDistance input; CA_active output; minDistances output
function [CA_active, minDistances] = collisionAvoidance(obstacleDistance)

persistent R_active;
if isempty(R_active)
    R_active = 5;
end

n = length(obstacleDistance);
CA_active = 0;
for i = 1:n
    if obstacleDistance <= R_active
        CA_active = 1;
    end
end

minAllowedDistToObstacle = ones(1,n)*0.3;

minDistances = minAllowedDistToObstacle;

%HARD CODED OVERRIDE BECAUSE THIS FUNCTIONALITY IS NOT SUFFICIENTLY
%IMPLEMENTED
%A method for supplying the CA system with a proper desired goal point has
%not been implemeted
CA_active = 0; %PATH FOLLOWING ONLY, i.e IGNORE OBSTACLES
%CA_active = 1; %CA SYSTEM ONLY, i.e IGNORE DESIRED PATH, goal point set in inverse kinematics block
%--------------
end

== matlab function USMcontrolSystem/Motion Control System/Kinematic Controller/Inverse Kinematics ==
  data: q input; pf_ref input; pr_ref input; g_joints_home input; T_I_f input; V_b_Ib_ref output; T_I_b input; T_I_r input; obstacleSurfacePoints input; CA_active input; qdot_ref output; modelParams parameter
function [V_b_Ib_ref, qdot_ref] = simulink_inverseKinematics(q, pf_ref, pr_ref, g_joints_home, T_I_f, T_I_b, T_I_r, obstacleSurfacePoints, CA_active, modelParams)
num_joints = modelParams.num_joints;
bodyTwists = modelParams.bodyTwists;
q_max = modelParams.q_max;
q_min = modelParams.q_min;

% Joint limit avoidance
% Calculating the normalized joint positions
q_normalized = (q - q_min)./(q_max - q_min);
alpha = 0.001;
W_jointLimit = alpha * (2*q_normalized - 1)./((1-q_normalized).^2 .* q_normalized.^2);

%% Calculate geometric Jacobians for the three points on the USM
%Calculate jacobian from base to end-effector
base = 2; %link number
sf = 2*base + 2; %Starting index for joint frames from base module and forward.
g_joints_home_f = g_joints_home(:,:,sf:end);
bodyTwists_f = bodyTwists(:, sf - 1:end);
num_joints_f = num_joints - 2*base;
Jf = calculateGeometricJacobian(g_joints_home_f, num_joints_f, bodyTwists_f);

%Calculate Jacobian from base to rear-end
eb = 2*base + 1; %Ending index for joint frames from base module and backward
num_joints_b = num_joints - num_joints_f;
g_joints_home_b = zeros(4,4,num_joints_b + 1);
for i = 1:eb
    g_joints_home_b(:,:,i) = g_joints_home(:,:, eb + 1 - i);
end
bodyTwists_b = fliplr(bodyTwists(:, 1:eb - 1));
Jr = calculateGeometricJacobian(g_joints_home_b, num_joints_b, bodyTwists_b);

%Calculate jacobian from base to base
Jb = [eye(6), zeros(6,4)];

%% Solve inverse kinematics
if CA_active == 1
    [V_b_Ib_ref, qdot_ref] = CLIK_collisionAvoidance(T_I_f, T_I_b, T_I_r, obstacleSurfacePoints, Jf, Jb, Jr);
else
    [qdot_ref] = CLIK_pathFollowing(Jf, Jr, T_I_f, T_I_r, pf_ref, pr_ref);
    V_b_Ib_ref = zeros(6,1);
end

end

== matlab function USMcontrolSystem/Data Logging/MATLAB Function ==
  data: rotm input; yaw output; pitch output; roll output
function [yaw,pitch,roll] = rotation2Euler(rotm)

eul = rotm2eul(rotm);

yaw = eul(1);
pitch = eul(2);
roll = eul(3);

end

== matlab function USMcontrolSystem/Vortex USM interface/Rear frame motion ==
  data: T_I_r output; R_I_r output; p_I_r output; T_I_vx input; T_vx_tail input; V_Ib_r output; T_tail_rear input; v_vx_tail input; omega_vx_tail input
function [T_I_r, R_I_r, p_I_r, V_Ib_r] = rearFrameMotion(T_I_vx, T_vx_tail, T_tail_rear, v_vx_tail, omega_vx_tail)
% Calculates the linear and angular velocity of the back frame relative to
% the inertial frame I, expressed in the back frame
% Assumption: No relative motion between the Vortex frame, F_vx, and the
% inertial frame, F_I

T_vx_b = T_vx_tail * T_tail_rear;
T_I_r = T_I_vx * T_vx_b;

R_vx_t = tform2rotm(T_vx_tail);
R_vx_b = tform2rotm(T_vx_b);
R_I_r = tform2rotm(T_I_r);
p_I_r = tform2trvec(T_I_r);


p_tb_t = tform2trvec(T_tail_rear);  % Vector from tail (t) to back (b) frame expressed in tail frame

v_Ib_b = R_vx_b' * (v_vx_tail + skew(omega_vx_tail) * R_vx_t * p_tb_t);
    
omega_Ib_b = R_vx_b' * omega_vx_tail;


V_Ib_r = [v_Ib_b; omega_Ib_b];

end

== matlab function USMcontrolSystem/Vortex USM interface/Front frame motion ==
  data: T_I_f output; R_I_f output; p_I_f output; T_I_vx input; T_vx_head input; V_If_f output; T_head_front input; v_vx_head input; omega_vx_head input
function [T_I_f, R_I_f, p_I_f, V_If_f] = frontFrameMotion(T_I_vx, T_vx_head, T_head_front, v_vx_head, omega_vx_head)
% Calculates the linear and angular velocity of the back frame relative to
% the inertial frame I, expressed in the back frame
% Assumption: No relative motion between the Vortex frame, F_vx, and the
% inertial frame, F_I

T_vx_f = T_vx_head * T_head_front;
T_I_f = T_I_vx * T_vx_f;

R_vx_h = tform2rotm(T_vx_head);
R_vx_f = tform2rotm(T_vx_f);
R_I_f = tform2rotm(T_I_f);
p_I_f = tform2trvec(T_I_f);


p_hf_h = tform2trvec(T_head_front);  % Vector from head (h) to front (f) frame expressed in head frame

v_If_f = R_vx_f' * (v_vx_head + skew(omega_vx_head) * R_vx_h * p_hf_h);
    
omega_If_f = R_vx_f' * omega_vx_head;


V_If_f = [v_If_f; omega_If_f];

end

== matlab function USMcontrolSystem/Vortex USM interface/Transformation matrix IC/Valid transform ==
  data: T input; valid output boolean
function valid = fcn(T)

valid = valid_tform(T);

== matlab function USMcontrolSystem/Vortex USM interface/Transformation matrix IC1/Valid transform ==
  data: T input; valid output boolean
function valid = fcn(T)

valid = valid_tform(T);

== matlab function USMcontrolSystem/Vortex USM interface/Base frame motion1 ==
  data: T_I_b output; R_I_b output; p_I_b output; T_I_vx input; T_vx_cm input; V_Ib_b output; T_cm_base input; v_vx_cm input; omega_vx_cm input
function [T_I_b, R_I_b, p_I_b, V_Ib_b] = baseFrameMotion(T_I_vx, T_vx_cm, T_cm_base, v_vx_cm, omega_vx_cm)
% Calculates the linear and angular velocity of the back frame relative to
% the inertial frame I, expressed in the back frame
% Assumption: No relative motion between the Vortex frame, F_vx, and the
% inertial frame, F_I

T_vx_b = T_vx_cm * T_cm_base;
T_I_b = T_I_vx * T_vx_b;

R_vx_c = tform2rotm(T_vx_cm);
R_vx_b = tform2rotm(T_vx_b);
R_I_b = tform2rotm(T_I_b);
p_I_b = tform2trvec(T_I_b);


p_cb_c = tform2trvec(T_cm_base);  % Vector from center module (c) to base (b) frame expressed in center module frame

v_Ib_b = R_vx_b' * (v_vx_cm + skew(omega_vx_cm) * R_vx_c * p_cb_c);
    
omega_Ib_b = R_vx_b' * omega_vx_cm;


V_Ib_b = [v_Ib_b; omega_Ib_b];

end

== matlab function USMcontrolSystem/Guidance System/3D WLOS ==
  data: waypoints input; V_b_Ib_tilde output; R_I_d output; T_I_b input; V_b_Ib input; delta parameter
function [V_b_Ib_tilde, R_I_d]  = simulink_WLOS(waypoints, T_I_b, V_b_Ib, delta)

[V_b_Ib_tilde, R_I_d] = WLOS(waypoints, T_I_b, V_b_Ib, delta);

end

== matlab function USMcontrolSystem/Motion Control System/Kinematic Controller/Forward Kinematics/Thruster configuration matrix ==
  data: g_thrusters input; TCM output; modelParams parameter
function TCM = thrusterConfiguration(g_thrusters, modelParams)
%#codegen

% Calculates the thruster configuration matrix in 6 DOF for the base frame
TCM = calculateTCM(g_thrusters,modelParams.num_thrusters);

end

== matlab function USMcontrolSystem/Vortex USM interface/MATLAB Function2 ==
  data: R input; eul output
function eul = rotation2Euler(R)

eul = rot2euler(R);

== matlab function USMcontrolSystem/Motion Control System/Dynamic Controller/Compute inertia matrix ==
  data: g_moduleCM input; M output; modelParams parameter
function M = inertiaMatrix(g_moduleCM, modelParams)
%#codegen

% g_moduleCM - homogeneous transformation matrices from base frame to CM of each module

num_modules = modelParams.num_modules;
mass = modelParams.mass;
addedMass = modelParams.addedMass(:,1:3);
momentOfInertia = modelParams.momentOfInertia;
addedInertia = modelParams.addedMass(:,4:6);

M = calculateInertiaMatrixRB(g_moduleCM, num_modules, mass, momentOfInertia, addedMass, addedInertia);

end

== matlab function USMcontrolSystem/Motion Control System/Dynamic Controller/Acceleration vector ==
  data: a_lin input; a output; a_ang input
function a = fcn(a_lin, a_ang)

a = [a_lin(1);a_lin(2);a_lin(3);a_ang(1);a_ang(2);a_ang(3)];
%a = [a1;0;0;0;0;a_ang];

== matlab function USMcontrolSystem/Guidance System/Configuration controller ==
  data: R_I_d input; pf_ref output; T_I_b input; pr_ref output; cf parameter
function [pf_ref, pr_ref] = simulink_configurationController(R_I_d, T_I_b, cf)

[pf_ref, pr_ref] = configurationController(R_I_d, T_I_b, cf);

end

== matlab function USMcontrolSystem/Vortex USM interface/Transformation matrix IC2/Valid transform ==
  data: T input; valid output boolean
function valid = fcn(T)

valid = valid_tform(T);

end
